simulink model "final_lqr_with_integral_controller"  (R2024a)
settings: Solver=VariableStepAuto  StartTime=0.0  StopTime=10.0  RelTol=1e-3
undefined symbols (not defined in the file): A_aug, B_aug, C_aug, D_aug, disturbance, g_val, Ki, Kx, m_val, r_pos
settings Model: Creator=yufon  LastModifiedBy=yufon

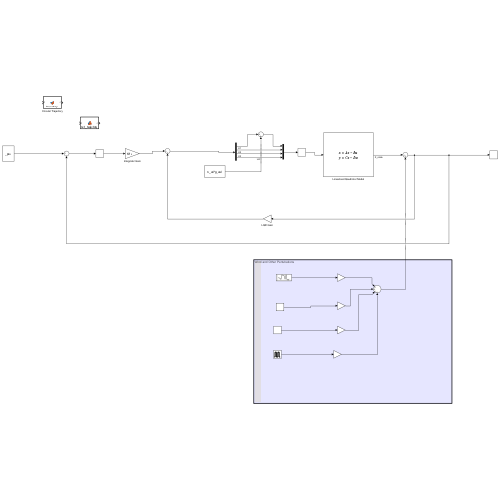
[thumbnail: Simulink's stored preview of the top-level diagram]
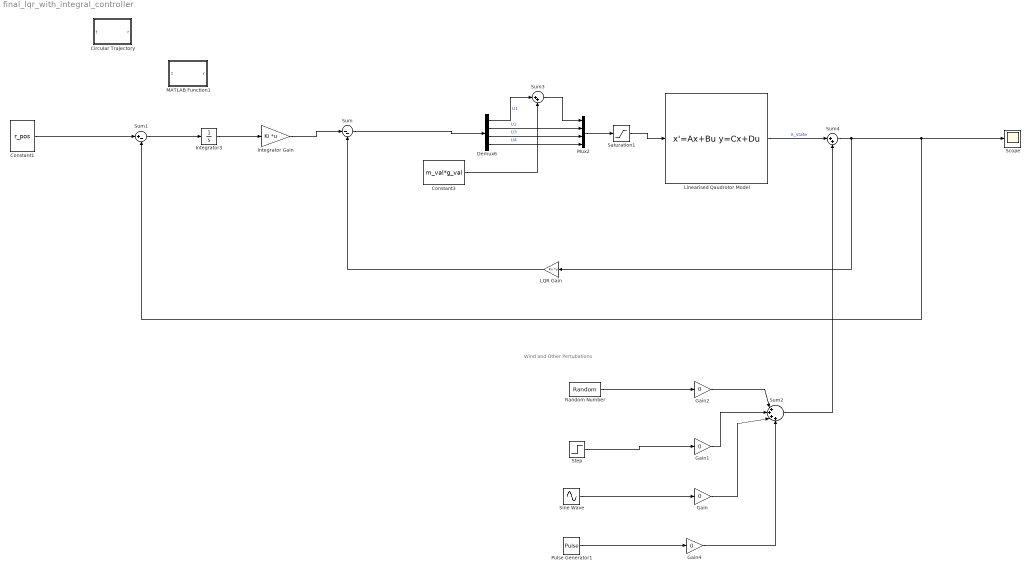
== system final_lqr_with_integral_controller ==
  note: Wind and Other Pertubations
  Circular Trajectory : MATLAB Function  TreatAsAtomicUnit=on
  Constant1 : Constant  Value=r_pos  VectorParams1D=off
  Constant3 : Constant  Value=m_val*g_val
  Demux6 : Demux
  Gain{,1..2,4} (4 alike) : Gain  Gain=0
  Integrator Gain : Gain  Gain=Ki  Multiplication=Matrix(K*u)
  Integrator3 : Integrator
  LQR Gain : Gain  Gain=Kx  Multiplication=Matrix(K*u)
  Linearised Qaudrotor Model : StateSpace  A=A_aug  B=B_aug  C=C_aug  D=D_aug  InitialCondition=0
  MATLAB Function1 : MATLAB Function  TreatAsAtomicUnit=on
  Mux2 : Mux
  Pulse Generator1 : DiscretePulseGenerator  PulseType=Time based  Period=10  PulseWidth=20  PhaseDelay=5
  Random Number : RandomNumber  Variance=0.5  SampleTime=0.1
  Saturation1 : Saturate  UpperLimit=[30; 0.15; 0.1; 0.5]  LowerLimit=[-3; -0.15; -0.1; -0.5]
  Scope : Scope
  Sine Wave : Sin  Frequency=0.5  SampleTime=0
  Step : Step  Before=zeros(12,1)  After=disturbance  SampleTime=0
  Sum : Sum  Inputs=|--
  Sum1 : Sum  Inputs=|+-
  Sum2 : Sum  Inputs=|++++
  Sum3 : Sum  Inputs=|++
  Sum4 : Sum  Inputs=|++
  wires:
  Gain1/1 -> Sum2/2
  Linearised Qaudrotor Model/1 -> Sum4/1  "X_state"
  Sum/1 -> Demux6/1
  Saturation1/1 -> Linearised Qaudrotor Model/1
  Integrator3/1 -> Integrator Gain/1
  Demux6/2 -> Mux2/2  "U2"
  Gain2/1 -> Sum2/1
  Mux2/1 -> Saturation1/1
  Integrator Gain/1 -> Sum/1
  Sum1/1 -> Integrator3/1
  Demux6/3 -> Mux2/3  "U3"
  Demux6/1 -> Sum3/1  "U1"
  Sum3/1 -> Mux2/1
  Sine Wave/1 -> Gain/1
  Random Number/1 -> Gain2/1
  Constant3/1 -> Sum3/2
  Constant1/1 -> Sum1/1
  Pulse Generator1/1 -> Gain4/1
  Gain/1 -> Sum2/3
  Step/1 -> Gain1/1
  Gain4/1 -> Sum2/4
  Sum2/1 -> Sum4/2
  Sum4/1 -> Scope/1, Sum1/2, LQR Gain/1
  Demux6/4 -> Mux2/4  "U4"
  LQR Gain/1 -> Sum/2

== matlab function final_lqr_with_integral_controller/MATLAB Function1 ==
  data: t input; r output
function r = rect_trajectory(t)

% Parameters
L = 10;        % Length of rectangle (x-direction)
W = 5;         % Width of rectangle (y-direction)
z0 = 10;       % Fixed height
T_side = 5;    % Time to complete one side
T_cycle = 4 * T_side;

% Normalize time to current phase
t_mod = mod(t, T_cycle);

% Initialize reference
x = 0;
y = 0;

if t_mod < T_side
    % Move right (+x)
    x = L * (t_mod / T_side);
    y = 0;

elseif t_mod < 2*T_side
    % Move forward (+y)
    x = L;
    y = W * ((t_mod - T_side) / T_side);

elseif t_mod < 3*T_side
    % Move left (−x)
    x = L - L * ((t_mod - 2*T_side) / T_side);
    y = W;

else
    % Move backward (−y)
    x = 0;
    y = W - W * ((t_mod - 3*T_side) / T_side);
end

% Fixed height
z = z0;

% Output as column vector
r = [x; y; z];

== matlab function final_lqr_with_integral_controller/Circular Trajectory ==
  data: t input; r output


function r = trajectory(t)

% Parameters (you can also pass these in or make them tunable)
R = 5;           % Radius of circle (meters)
omega = 0.1;     % Angular frequency (rad/s)
z0 = 10;         % Base altitude (meters)
A = 2;           % Amplitude of vertical oscillation (meters)
omega_z = 0.05;  % Vertical oscillation frequency (rad/s)

% Reference trajectory components
r_x = R * cos(omega * t);
r_y = R * sin(omega * t);
r_z = z0 + A * sin(omega_z * t);  % Set A = 0 for pure circle

% Output as a 3x1 vector
r = [r_x; r_y; r_z];
